simulink model "Model_based_Controller"  (R2020a)
settings: Solver=VariableStepAuto  StartTime=0.0  StopTime=10.0  FixedStep=0.005  RelTol=1e-3
values from neighbouring files (symbols this model uses):
  F = [f1 , 0 ... (first row only)    [parameters.m]
  Kd = [10, 0 ... (first row only)    [parameters.m]
  Kp = [30 , 0 ... (first row only)    [parameters.m]
settings Model: Creator=sirius  LastModifiedBy=sirius

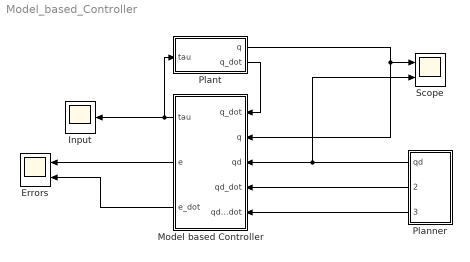
== system Model_based_Controller ==
  Errors : Scope  NumInputPorts=2
  Input : Scope
  Model based Controller : Subsystem
  Planner : Subsystem
  Plant : Subsystem
  Scope : Scope  NumInputPorts=2
  wires:
  Plant/1(q) -> Model based Controller/2(q), Scope/1
  Planner/1(qd) -> Model based Controller/3(qd), Scope/2
  Model based Controller/1(tau) -> Input/1, Plant/1(tau)
  Plant/2(q_dot) -> Model based Controller/1(q_dot)
  Planner/2(qd_dot) -> Model based Controller/4(qd_dot)
  Planner/3(qd_ddot) -> Model based Controller/5(qd_ddot)
  Model based Controller/2(e) -> Errors/1
  Model based Controller/3(e_dot) -> Errors/2

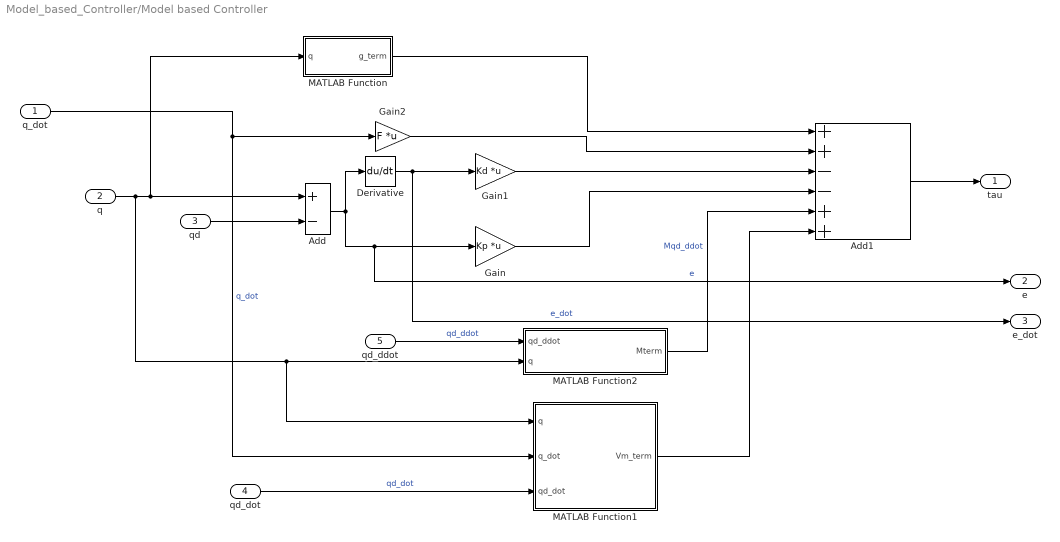
== system Model_based_Controller/Model based Controller ==
  q_dot : Inport
  q : Inport  Port=2
  qd : Inport  Port=3
  qd_dot : Inport  Port=4
  qd_ddot : Inport  Port=5
  Add : Sum  Inputs=+-
  Add1 : Sum  Inputs=++--++
  Derivative : Derivative
  Gain : Gain  Gain=Kp  Multiplication=Matrix(K*u)
  Gain1 : Gain  Gain=Kd  Multiplication=Matrix(K*u)
  Gain2 : Gain  Gain=F  Multiplication=Matrix(K*u)
  MATLAB Function : MATLAB Function  TreatAsAtomicUnit=on
  MATLAB Function1 : MATLAB Function  TreatAsAtomicUnit=on
  MATLAB Function2 : MATLAB Function  TreatAsAtomicUnit=on
  tau : Outport
  e : Outport  Port=2
  e_dot : Outport  Port=3
  wires:
  q/1 -> MATLAB Function1/1(q), MATLAB Function2/2(q), Add/1, MATLAB Function/1(q)
  Add/1 -> e/1, Gain/1, Derivative/1  "e"
  Derivative/1 -> e_dot/1, Gain1/1  "e_dot"
  Add1/1 -> tau/1
  qd/1 -> Add/2
  qd_dot/1 -> MATLAB Function1/3(qd_dot)  "qd_dot"
  qd_ddot/1 -> MATLAB Function2/1(qd_ddot)  "qd_ddot"
  q_dot/1 -> MATLAB Function1/2(q_dot), Gain2/1  "q_dot"
  Gain/1 -> Add1/4
  Gain1/1 -> Add1/3
  Gain2/1 -> Add1/2
  MATLAB Function/1(g_term) -> Add1/1
  MATLAB Function1/1(Vm_term) -> Add1/6
  MATLAB Function2/1(Mterm) -> Add1/5  "Mqd_ddot"

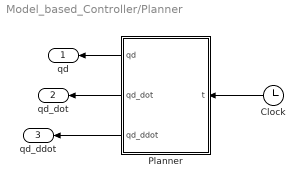
== system Model_based_Controller/Planner ==
  Clock : Clock
  Planner : MATLAB Function  TreatAsAtomicUnit=on
  qd : Outport
  qd_dot : Outport  Port=2
  qd_ddot : Outport  Port=3
  wires:
  Clock/1 -> Planner/1(t)
  Planner/1(qd) -> qd/1
  Planner/2(qd_dot) -> qd_dot/1
  Planner/3(qd_ddot) -> qd_ddot/1

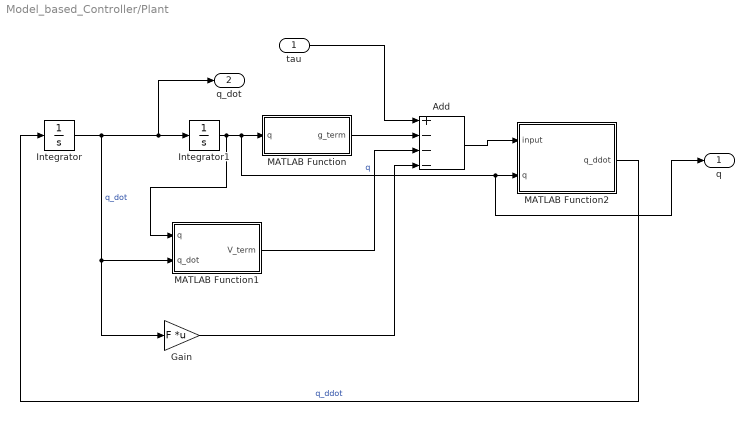
== system Model_based_Controller/Plant ==
  tau : Inport
  Add : Sum  Inputs=+---
  Gain : Gain  Gain=F  Multiplication=Matrix(K*u)
  Integrator : Integrator  InitialCondition=[0;0]
  Integrator1 : Integrator  InitialCondition=[0;0]
  MATLAB Function : MATLAB Function  TreatAsAtomicUnit=on
  MATLAB Function1 : MATLAB Function  TreatAsAtomicUnit=on
  MATLAB Function2 : MATLAB Function  TreatAsAtomicUnit=on
  q : Outport
  q_dot : Outport  Port=2
  wires:
  MATLAB Function2/1(q_ddot) -> Integrator/1  "q_ddot"
  MATLAB Function/1(g_term) -> Add/2
  Add/1 -> MATLAB Function2/1(input)
  MATLAB Function1/1(V_term) -> Add/3
  Integrator/1 -> Gain/1, MATLAB Function1/2(q_dot), q_dot/1, Integrator1/1  "q_dot"
  tau/1 -> Add/1
  Gain/1 -> Add/4
  Integrator1/1 -> MATLAB Function1/1(q), q/1, MATLAB Function2/2(q), MATLAB Function/1(q)  "q"

== matlab function Model_based_Controller/Plant/MATLAB Function ==
  data: q input; g_term output
function g_term = G(q)
g_term = [35.9929*cos(q(1)) + 1.92276*cos(q(1) + q(2));
          1.92276*cos(q(1) + q(2));];

== matlab function Model_based_Controller/Plant/MATLAB Function2 ==
  data: input input; q_ddot output; q input
function q_ddot = M_inverse(input,q)
M = [ 0.3920*cos(q(2)) + 3.8650, 0.196*cos(q(2)) + 0.196;
   0.196*cos(q(2)) + 0.196,                    0.196;];
q_ddot = M\input;
end

== matlab function Model_based_Controller/Planner/Planner ==
  data: t input; qd output; qd_dot output; qd_ddot output
function [qd,qd_dot,qd_ddot] = Traj(t)
qd = [pi/3 + pi/6*sin(t);
      pi/4 + pi/6*cos(t)];

qd_dot = [-pi/6*cos(t);
          pi/6*sin(t);];
qd_ddot = [-pi/6*sin(t);
           -pi/6*cos(t);];

== matlab function Model_based_Controller/Model based Controller/MATLAB Function ==
  data: q input; g_term output
function g_term = G(q)
g_term = [35.9929*cos(q(1)) + 1.92276*cos(q(1) + q(2));
          1.92276*cos(q(1) + q(2));];
end

== matlab function Model_based_Controller/Model based Controller/MATLAB Function2 ==
  data: qd_ddot input; Mterm output; q input
function Mterm = M(qd_ddot,q)
M = [ 0.3920*cos(q(2)) + 3.8650, 0.196*cos(q(2)) + 0.196;
   0.196*cos(q(2)) + 0.196,                    0.196;];
Mterm = M*qd_ddot;
end

== matlab function Model_based_Controller/Model based Controller/MATLAB Function1 ==
  data: q input; Vm_term output; q_dot input; qd_dot input
function Vm_term = Vm(q,q_dot,qd_dot)
Vm_Mat = [ -0.196*q_dot(2)*sin(q(2)), -0.196*sin(q(2))*(q_dot(1) + q_dot(2));
            0.196*q_dot(1)*sin(q(2)),                           0];
Vm_term = Vm_Mat*qd_dot;
end

== matlab function Model_based_Controller/Plant/MATLAB Function1 ==
  data: q input; V_term output; q_dot input
function V_term = V(q,q_dot)

V_term = [-0.196*(2*q_dot(1)*q_dot(2) + q_dot(2)^2)*sin(q(2));
            0.196*(q_dot(1)^2)*sin(q(2))];
end
